simulink model "ModeInputHandle"  (R2018b)
settings: Solver=FixedStepDiscrete  StartTime=0.0  StopTime=10.0  FixedStep=0.01  RelTol=1e-3
undefined symbols (not defined in the file or in its folder): c, CmprtMdHMIReqExt2Tp1, CmprtMdHMIReqExtTp1, CmprtMdHMIReqTp1, d, e, EZESwReq1, f, g, IfVeSMSeStNumConfig, j, KeSMSuButtonLongPressedThrshldTm_Val, KeSMSuFoldType_Val, KeSMSwSeatSMSSeatMdTrigGapTimer_Val, KeSMSwSeatTrigWaitTimer_Val, KeSMSwSRSActiveValidTm_Val, LckUlckActvtFunc1, LstLckFunc1, LugSelectSw1, MdReqTp1, PowerMode1, SeatOccupiedSts1, SRSMode1, StPassCmprtMdCtrl_Md10_VCUConfig_Val, StPassCmprtMdCtrl_Md11_VCUConfig_Val, StPassCmprtMdCtrl_Md12_VCUConfig_Val, StPassCmprtMdCtrl_Md13_VCUConfig_Val, StPassCmprtMdCtrl_Md1_VCUConfig_Val, StPassCmprtMdCtrl_Md27_VCUConfig_Val, StPassCmprtMdCtrl_Md28_VCUConfig_Val, StPassCmprtMdCtrl_Md29_VCUConfig_Val, StPassCmprtMdCtrl_Md2_VCUConfig_Val, StPassCmprtMdCtrl_Md30_VCUConfig_Val, StPassCmprtMdCtrl_Md31_VCUConfig_Val, StPassCmprtMdCtrl_Md32_VCUConfig_Val, StPassCmprtMdCtrl_Md3_VCUConfig_Val, StPassCmprtMdCtrl_Md53_VCUConfig_Val, StPassCmprtMdCtrl_Md56_VCUConfig_Val, StPassCmprtMdCtrl_Md57_VCUConfig_Val, StPassCmprtMdCtrl_Md58_VCUConfig_Val, StPassCmprtMdCtrl_Md61_VCUConfig_Val, StPassCmprtMdCtrl_Md62_VCUConfig_Val, StPassCmprtMdCtrl_Md8_VCUConfig_Val, StPassCmprtMdCtrl_Md9_VCUConfig_Val, StSrv_StMd10_Config_Val, StSrv_StMd11_Config_Val, StSrv_StMd12_Config_Val, StSrv_StMd13_Config_Val, StSrv_StMd1_Config_Val, StSrv_StMd27_Config_Val, StSrv_StMd28_Config_Val, StSrv_StMd29_Config_Val, StSrv_StMd2_Config_Val, StSrv_StMd30_Config_Val, StSrv_StMd31_Config_Val, StSrv_StMd32_Config_Val, StSrv_StMd3_Config_Val, StSrv_StMd8_Config_Val, StSrv_StMd9_Config_Val, VehMovState1
libraries: MSMLib x91
(part 8 of 9)

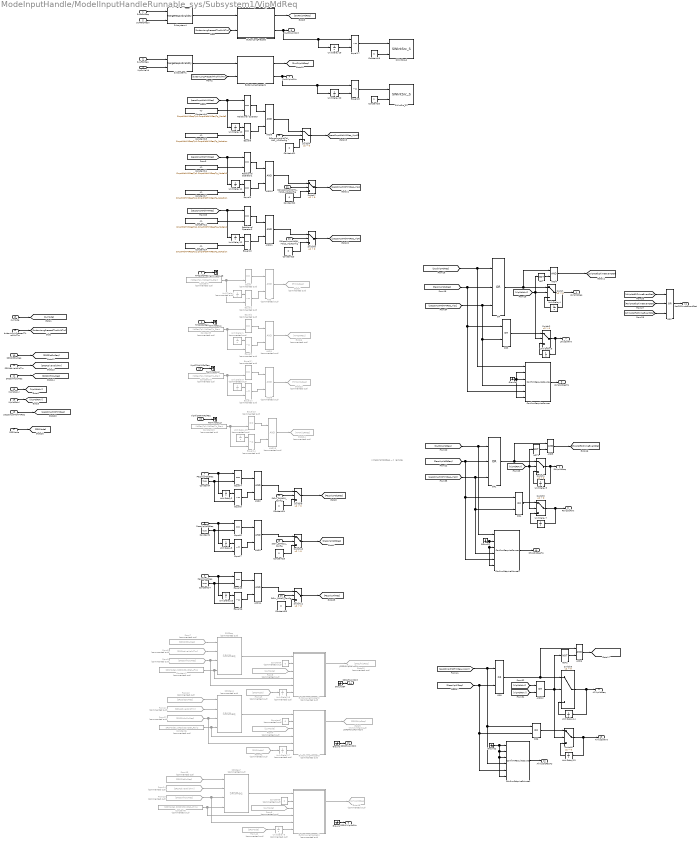
== system ModeInputHandle/ModelInputHandleRunnable_sys/Subsystem1/VipMdReq ==
  note: //SRSLfVipRclIntCnt
  note: // PassVipMdLtReq ---》 remote
  note: //SRSRtVipRclIntCnt
  SwRtRclReq : Inport
  SwRtRclReqV : Inport  Port=2
  SwLfRclReq : Inport  Port=3
  VipSwValid : Inport  Port=4
  HMI2LRclReq : Inport  Port=5
  HMI2RRclReq : Inport  Port=6
  PassVipMdLtReq : Inport  Port=7
  PassVipMdRtReq : Inport  Port=8
  PassVipAllReq : Inport  Port=9
  SRSSlctSwReq : Inport  Port=10
  SRSCnfmSwReq : Inport  Port=11
  buttonLongPressedThrshhldTm : Inport  Port=12
  curMode : Inport  Port=13
  SRSActiveValidTm : Inport  Port=14
  VipMdLtAvl : Inport  Port=15
  VipMdRtAvl : Inport  Port=16
  SRSMode : Inport  Port=17
  passCmprtMdHMIReq : Inport  Port=18
  VipAll2LHMIRclReq : Inport  Port=19
  VipAll2RHMIRclReq : Inport  Port=20
  StPassCmprtMdCtrl_Md10_VCUConfig : Inport  Port=21
  StPassCmprtMdCtrl_Md12_VCUConfig : Inport  Port=22
  StPassCmprtMdCtrl_Md2_VCUConfig : Inport  Port=23
  StSrv_StMd10_Config : Inport  Port=24
  StSrv_StMd12_Config : Inport  Port=25
  StSrv_StMd2_Config : Inport  Port=26
  AND{,1,8,13} (4 alike) : Logic  Commented=on  AllPortsSameDT=off  OutDataTypeStr=boolean
  AND{2..6,9..11,14} (9 alike) : Logic  AllPortsSameDT=off  OutDataTypeStr=boolean
  AND12 : Logic  Operator=OR  AllPortsSameDT=off  OutDataTypeStr=boolean
  ButtonLongPressed : Subsystem  AncestorBlock=MSMLib/ButtonLongPressed
  ButtonLongPressed1 : Subsystem  AncestorBlock=MSMLib/ButtonLongPressed
  ButtonLongPressed2 : Subsystem  Commented=on  AncestorBlock=MSMLib/ButtonLongPressed
  ButtonLongPressed3 : Subsystem  Commented=on  AncestorBlock=MSMLib/ButtonLongPressed
  ButtonLongPressed4 : Subsystem  Commented=on  AncestorBlock=MSMLib/ButtonLongPressed
  ConfirmRequireSource : MSMLib/ConfirmRequireSource  SystemSampleTime=-1
  ConfirmRequireSource1 : MSMLib/ConfirmRequireSource  SystemSampleTime=-1
  ConfirmRequireSource2 : MSMLib/ConfirmRequireSource  SystemSampleTime=-1
  Constant{,3,13,16} (4 alike) : Constant  Commented=on  Value=MdReqTp1.MdReqTp_Start
  Constant1 : Constant  Value=true  OutDataTypeStr=boolean
  Constant10 : Constant  Value=CmprtMdHMIReqTp1.CmprtMdHMIReqTp_Mode2  OutDataTypeStr=Enum:CmprtMdHMIReqTp1
  Constant11 : Constant  Value=CmprtMdHMIReqTp1.CmprtMdHMIReqTp_Mode10  OutDataTypeStr=Enum:CmprtMdHMIReqTp1
  Constant12 : Constant  Value=CmprtMdHMIReqTp1.CmprtMdHMIReqTp_Mode12  OutDataTypeStr=Enum:CmprtMdHMIReqTp1
  Constant14 : Constant  Value=true  OutDataTypeStr=boolean
  Constant15 : Constant  Value=CmprtMdHMIReqTp1.CmprtMdHMIReqTp_NoAction  OutDataTypeStr=Enum:CmprtMdHMIReqTp1
  Constant17 : Constant  Value=CmprtMdHMIReqTp1.CmprtMdHMIReqTp_NoAction  OutDataTypeStr=Enum:CmprtMdHMIReqTp1
  Constant18 : Constant  Value=CmprtMdHMIReqTp1.CmprtMdHMIReqTp_NoAction  OutDataTypeStr=Enum:CmprtMdHMIReqTp1
  Constant19 : Constant  Value=3  OutDataTypeStr=uint8
  Constant2 : Constant  Commented=on  Value=SRSMode1.SRSSlctSwStat_LfVip  OutDataTypeStr=Enum:SRSMode1
  Constant20 : Constant  Value=2  OutDataTypeStr=uint8
  Constant{21..26} (6 alike) : Constant  Value=0  VectorParams1D=off  OutDataTypeStr=boolean  SampleTime=-1
  Constant4 : Constant  Value=true  OutDataTypeStr=boolean
  Constant5 : Constant  Commented=on  Value=0  OutDataTypeStr=uint8
  Constant6 : Constant  Commented=on  Value=SRSMode1.SRSSlctSwStat_RtVip  OutDataTypeStr=Enum:SRSMode1
  Constant7 : Constant  Commented=on  Value=0  OutDataTypeStr=uint8
  Constant8 : Constant  Commented=on  Value=SRSMode1.SRSSlctSwStat_AllVip  OutDataTypeStr=Enum:SRSMode1
  Constant9 : Constant  Commented=on  Value=0  OutDataTypeStr=uint8
  Equal{,2,11,13} (4 alike) : RelationalOperator  Commented=on  Operator===  OutDataTypeStr=boolean  RndMeth=Simplest
  Equal{1,3,12,14} (4 alike) : RelationalOperator  Commented=on  Operator=~=  OutDataTypeStr=boolean  RndMeth=Simplest
  Equal{4,6,8..10,15} (6 alike) : RelationalOperator  Operator===  OutDataTypeStr=boolean  RndMeth=Simplest
  Equal{5,7,16..18} (5 alike) : RelationalOperator  Operator=~=  OutDataTypeStr=boolean  RndMeth=Simplest
  From10 : From  Commented=on  GotoTag=SRSSlctSwReq
  From11 : From  Commented=on  GotoTag=SRSActiveValidTm
  From12 : From  Commented=on  GotoTag=SRSCnfmSwReq
  From13 : From  Commented=on  GotoTag=SRSSlctSwReq
  From14 : From  Commented=on  GotoTag=SRSActiveValidTm
  From15 : From  Commented=on  GotoTag=SRSCnfmSwReq
  From4 : From  Commented=on  GotoTag=curMode
  From40 : From  Commented=on  GotoTag=SRSMode
  From42 : From  Commented=on  GotoTag=SRSMode
  From43 : From  Commented=on  GotoTag=SRSMode
  From5 : From  Commented=on  GotoTag=curMode
  From6 : From  Commented=on  GotoTag=curMode
  From7 : From  Commented=on  GotoTag=SRSSlctSwReq
  From8 : From  Commented=on  GotoTag=SRSActiveValidTm
  From9 : From  Commented=on  GotoTag=SRSCnfmSwReq
  Goto10 : Goto  Commented=on  GotoTag=SRSLfVipReq
  Goto18 : Goto  Commented=on  GotoTag=AllVipMdReq
  Goto23 : Goto  Commented=on  GotoTag=HMIAll2LReq
  Goto24 : Goto  Commented=on  GotoTag=HMIAll2RReq
  Goto6 : Goto  Commented=on  GotoTag=HMI2RReq
  Goto7 : Goto  Commented=on  GotoTag=HMI2LReq
  Goto9 : Goto  Commented=on  GotoTag=SRSRtVipReq
  Ground{,1..4,84} (6 alike) : Ground
  NOT : Logic  Operator=NOT  AllPortsSameDT=off  OutDataTypeStr=boolean
  NOT1 : Logic  Operator=NOT  AllPortsSameDT=off  OutDataTypeStr=boolean
  NOT2 : Logic  Operator=NOT  AllPortsSameDT=off  OutDataTypeStr=boolean
  OR : Logic  Operator=OR  Inputs=3  AllPortsSameDT=off  OutDataTypeStr=boolean
  OR1 : Logic  Operator=OR  Inputs=3  AllPortsSameDT=off  OutDataTypeStr=boolean
  OR2 : Logic  Operator=OR  Inputs=3  AllPortsSameDT=off  OutDataTypeStr=boolean
  OR{3..6} (4 alike) : Logic  Operator=OR  AllPortsSameDT=off  OutDataTypeStr=boolean
  Relational Operator : RelationalOperator  Operator===  OutDataTypeStr=boolean  RndMeth=Simplest
  Relational Operator1 : RelationalOperator  Operator===  OutDataTypeStr=boolean  RndMeth=Simplest
  Relational Operator2 : RelationalOperator  Operator===  OutDataTypeStr=boolean  RndMeth=Simplest
  SRSReq : MSMLib/SRSReq  Commented=on  SystemSampleTime=-1
  SRSReq1 : MSMLib/SRSReq  Commented=on  SystemSampleTime=-1
  SRSReq2 : MSMLib/SRSReq  Commented=on  SystemSampleTime=-1
  SWIntSrc_S : MSMLib/SWIntSrc_S  SystemSampleTime=-1
  SWIntSrc_S1 : MSMLib/SWIntSrc_S  SystemSampleTime=-1
  Subsystem1 : MSMLib/MergeReqAndValidity  SystemSampleTime=-1
  Subsystem4 : MSMLib/MergeReqAndValidity  SystemSampleTime=-1
  Switch{,1..11} (12 alike) : Switch  Criteria=u2 > Threshold
  Terminator_{1..3,69} (4 alike) : Terminator
  Unit Delay{,1,9,15} (4 alike) : UnitDelay  Commented=on  InitialCondition=e  SampleTime=-1
  Unit Delay10 : UnitDelay  InitialCondition=c  SampleTime=-1
  Unit Delay11 : UnitDelay  InitialCondition=c  SampleTime=-1
  Unit Delay12 : UnitDelay  InitialCondition=c  SampleTime=-1
  Unit Delay{2..7,13..14,16,19..20} (11 alike) : UnitDelay  SampleTime=-1
  Unit Delay17 : UnitDelay  Commented=on  InitialCondition=d  SampleTime=-1
  Unit Delay18 : UnitDelay  Commented=on  InitialCondition=d  SampleTime=-1
  Unit Delay8 : UnitDelay  Commented=on  InitialCondition=d  SampleTime=-1
  LtVipMdReq : Outport
  RtVipMdReq : Outport  Port=2
  AllVipMdReq : Outport  Port=3
  SwLfVipIntCnt : Outport  Port=4
  SwRtVipIntCnt : Outport  Port=5
  SRSAllVipIntCnt : Outport  Port=6
  LtVipSoftInt : Outport  Port=7
  RtVipSoftInt : Outport  Port=8
  "LtVipSrcReqTp " : Outport  Port=9
  "RtVipSrcReqTp " : Outport  Port=10
  Notf1ChimeEventStat : Outport  Port=11
  AllVipSrcReqTp : Outport  Port=12
  AllVipSoftInt : Outport  Port=13
  SRSLfVipIntCnt : Outport  Port=14
  SRSRtVipIntCnt : Outport  Port=15
  wires:
  buttonLongPressedThrshhldTm/1 -> [buttonLongPressedThrshhldTm]
  curMode/1 -> [curMode]
  SwRtRclReqV/1 -> Subsystem4/2
  [buttonLongPressedThrshhldTm] -> ButtonLongPressed1/2(longPressThrshhldTm)
  [buttonLongPressedThrshhldTm] -> ButtonLongPressed/2(longPressThrshhldTm)
  SwRtRclReq/1 -> Subsystem4/1
  Subsystem4/1 -> ButtonLongPressed/1(modeReq)
  Equal2/1 -> AND1/1
  Equal1/1 -> AND/2
  AND/1 -> Goto7/1
  Equal/1 -> AND/1
  AND1/1 -> Goto6/1
  Constant3/1 -> Equal3/2, Equal2/2
  Equal3/1 -> AND1/2
  Unit Delay/1 -> Equal1/1
  Unit Delay1/1 -> Equal3/1
  Constant/1 -> Equal1/2, Equal/2
  Constant4/1 -> Equal4/2, Equal5/2
  PassVipMdLtReq/1 -> Unit Delay2/1, Equal4/1
  Equal4/1 -> AND2/1
  Unit Delay2/1 -> Equal5/1
  Equal5/1 -> AND2/2
  Equal7/1 -> AND3/2
  Equal6/1 -> AND3/1
  Unit Delay3/1 -> Equal7/1
  Constant1/1 -> Equal6/2, Equal7/2
  PassVipMdRtReq/1 -> Unit Delay3/1, Equal6/1
  SRSReq/1 -> ButtonLongPressed2/1(modeReq)
  Constant2/1 -> ButtonLongPressed2/4(CmpReq), SRSReq/4
  From5/1 -> ButtonLongPressed2/3(curMdState)
  Constant5/1 -> ButtonLongPressed2/2(longPressThrshhldTm)
  ButtonLongPressed2/1(mdReq) -> Goto10/1
  From4/1 -> ButtonLongPressed3/3(curMdState)
  ButtonLongPressed3/1(mdReq) -> Goto9/1
  SRSReq1/1 -> ButtonLongPressed3/1(modeReq)
  Constant6/1 -> ButtonLongPressed3/4(CmpReq), SRSReq1/4
  Constant7/1 -> ButtonLongPressed3/2(longPressThrshhldTm)
  From6/1 -> ButtonLongPressed4/3(curMdState)
  SRSReq2/1 -> ButtonLongPressed4/1(modeReq)
  Constant8/1 -> ButtonLongPressed4/4(CmpReq), SRSReq2/4
  Constant9/1 -> ButtonLongPressed4/2(longPressThrshhldTm)
  SRSSlctSwReq/1 -> [SRSSlctSwReq]
  SRSActiveValidTm/1 -> [SRSActiveValidTm]
  SRSCnfmSwReq/1 -> [SRSCnfmSwReq]
  From7/1 -> SRSReq/1
  From8/1 -> SRSReq/2
  From9/1 -> ButtonLongPressed2/5(SRSCnfmSwReq), SRSReq/3
  From12/1 -> ButtonLongPressed3/5(SRSCnfmSwReq), SRSReq1/3
  From11/1 -> SRSReq1/2
  From10/1 -> SRSReq1/1
  From15/1 -> ButtonLongPressed4/5(SRSCnfmSwReq), SRSReq2/3
  From14/1 -> SRSReq2/2
  From13/1 -> SRSReq2/1
  ButtonLongPressed/1(mdReq) -> [SwRtVipMdReq]
  ButtonLongPressed1/1(mdReq) -> [SwLfVipMdReq]
  [SwLfVipMdReq] -> OR/1, ConfirmRequireSource/1
  [PassVipMdLtReq] -> OR/2, OR3/1, ConfirmRequireSource/5
  [SwRtVipMdReq] -> OR1/1, ConfirmRequireSource1/1
  [PassVipMdRtReq] -> OR1/2, ConfirmRequireSource1/5, OR4/1
  ConfirmRequireSource/1 -> "LtVipSrcReqTp "/1
  ConfirmRequireSource1/1 -> "RtVipSrcReqTp "/1
  [VipMdLtAvl] -> Switch/2, NOT/1, Switch2/2
  OR/1 -> AND4/1, Switch/1
  Switch/1 -> Unit Delay4/1, LtVipMdReq/1
  Unit Delay4/1 -> Switch/3
  [VipMdRtAvl] -> Switch3/2, NOT1/1, Switch1/2
  OR1/1 -> AND5/1, Switch1/1
  Switch1/1 -> Unit Delay5/1, RtVipMdReq/1
  Unit Delay5/1 -> Switch1/3
  NOT/1 -> AND4/2
  AND4/1 -> [LtVipNotf1ChimeEventStat]
  NOT1/1 -> AND5/2
  AND5/1 -> [RtVipNotf1ChimeEventStat]
  VipMdLtAvl/1 -> [VipMdLtAvl]
  VipMdRtAvl/1 -> [VipMdRtAvl]
  [LtVipNotf1ChimeEventStat] -> OR2/1
  [RtVipNotf1ChimeEventStat] -> OR2/2
  [AllVipNotf1ChimeEventStat] -> OR2/3
  OR2/1 -> Notf1ChimeEventStat/1
  Switch2/1 -> LtVipSoftInt/1, Unit Delay6/1
  Unit Delay6/1 -> Switch2/3
  OR3/1 -> Switch2/1
  Switch3/1 -> RtVipSoftInt/1, Unit Delay7/1
  Unit Delay7/1 -> Switch3/3
  OR4/1 -> Switch3/1
  ButtonLongPressed4/1(mdReq) -> Goto18/1
  Ground/1 -> ConfirmRequireSource/6, ConfirmRequireSource/2, ConfirmRequireSource/3
  Unit Delay8/1 -> ButtonLongPressed4/6(SRSMode)
  Ground1/1 -> ConfirmRequireSource1/6, ConfirmRequireSource1/3, ConfirmRequireSource1/2
  Constant10/1 -> Relational Operator/2
  [passCmprtMdHMIReq] -> Unit Delay10/1, Relational Operator/1
  Equal8/1 -> AND9/2
  Unit Delay10/1 -> Equal8/1
  Relational Operator/1 -> AND9/1
  passCmprtMdHMIReq/1 -> [passCmprtMdHMIReq]
  Equal9/1 -> AND10/2
  Constant11/1 -> Relational Operator1/2
  Relational Operator1/1 -> AND10/1
  [passCmprtMdHMIReq] -> Unit Delay11/1, Relational Operator1/1
  Unit Delay11/1 -> Equal9/1
  Relational Operator2/1 -> AND11/1
  [passCmprtMdHMIReq] -> Unit Delay12/1, Relational Operator2/1
  Unit Delay12/1 -> Equal10/1
  Equal10/1 -> AND11/2
  Constant12/1 -> Relational Operator2/2
  [passCmprtMdHMIReq_VipL] -> OR/3, ConfirmRequireSource/4, OR3/2
  [passCmprtMdHMIReq_VipR] -> ConfirmRequireSource1/4, OR4/2, OR1/3
  [passCmprtMdHMIReq_VipAll] -> OR5/1, ConfirmRequireSource2/4, OR6/1
  ConfirmRequireSource2/1 -> AllVipSrcReqTp/1
  Unit Delay13/1 -> Switch6/3
  Switch5/1 -> Unit Delay14/1, AllVipMdReq/1
  Switch6/1 -> AllVipSoftInt/1, Unit Delay13/1
  Unit Delay14/1 -> Switch5/3
  AND12/1 -> Switch6/2, NOT2/1, Switch5/2
  OR5/1 -> Switch5/1, AND6/1
  [VipMdLtAvl] -> AND12/1
  [VipMdRtAvl] -> AND12/2
  AND8/1 -> Goto23/1
  Equal11/1 -> AND8/1
  Equal12/1 -> AND8/2
  Constant16/1 -> Equal12/2, Equal11/2
  Unit Delay9/1 -> Equal12/1
  OR6/1 -> Switch6/1
  Equal14/1 -> AND13/2
  Unit Delay15/1 -> Equal14/1
  Equal13/1 -> AND13/1
  AND13/1 -> Goto24/1
  Constant13/1 -> Equal14/2, Equal13/2
  Equal15/1 -> AND14/1
  Constant14/1 -> Equal15/2, Equal16/2
  Equal16/1 -> AND14/2
  Unit Delay16/1 -> Equal16/1
  PassVipAllReq/1 -> Unit Delay16/1, Equal15/1
  [PassVipAllReq] -> OR5/2, OR6/2, ConfirmRequireSource2/5
  ButtonLongPressed/2(mdInterruptCnt) -> Unit Delay19/1, Equal17/1, SwRtVipIntCnt/1
  ButtonLongPressed1/2(mdInterruptCnt) -> Unit Delay20/1, Equal18/1, SwLfVipIntCnt/1
  Subsystem1/1 -> ButtonLongPressed1/1(modeReq)
  VipSwValid/1 -> Subsystem1/2
  SwLfRclReq/1 -> Subsystem1/1
  SRSMode/1 -> [SRSMode]
  From40/1 -> Unit Delay8/1
  From42/1 -> Unit Delay17/1
  Unit Delay17/1 -> ButtonLongPressed3/6(SRSMode)
  From43/1 -> Unit Delay18/1
  Unit Delay18/1 -> ButtonLongPressed2/6(SRSMode)
  NOT2/1 -> AND6/2
  AND6/1 -> [AllVipNotf1ChimeEventStat]
  Constant15/1 -> Equal8/2
  Constant17/1 -> Equal9/2
  Constant18/1 -> Equal10/2
  Unit Delay19/1 -> Equal17/2
  Equal17/1 -> SWIntSrc_S/1
  Constant19/1 -> SWIntSrc_S/2
  Unit Delay20/1 -> Equal18/2
  Equal18/1 -> SWIntSrc_S1/1
  Constant20/1 -> SWIntSrc_S1/2
  HMI2LRclReq/1 -> Terminator_69/1
  HMI2RRclReq/1 -> Terminator_1/1
  VipAll2LHMIRclReq/1 -> Terminator_2/1
  VipAll2RHMIRclReq/1 -> Terminator_3/1
  Ground84/1 -> SRSLfVipIntCnt/1
  Ground3/1 -> SRSRtVipIntCnt/1
  Ground4/1 -> SRSAllVipIntCnt/1
  Ground2/1 -> ConfirmRequireSource2/6, ConfirmRequireSource2/3, ConfirmRequireSource2/2, ConfirmRequireSource2/1
  StPassCmprtMdCtrl_Md2_VCUConfig/1 -> Switch4/2
  Constant21/1 -> Switch4/3
  Switch4/1 -> [passCmprtMdHMIReq_VipAll]
  AND9/1 -> Switch4/1
  StPassCmprtMdCtrl_Md10_VCUConfig/1 -> Switch7/2
  AND10/1 -> Switch7/1
  Switch7/1 -> [passCmprtMdHMIReq_VipL]
  Constant22/1 -> Switch7/3
  StPassCmprtMdCtrl_Md12_VCUConfig/1 -> Switch8/2
  AND11/1 -> Switch8/1
  Constant23/1 -> Switch8/3
  Switch8/1 -> [passCmprtMdHMIReq_VipR]
  StSrv_StMd10_Config/1 -> Switch9/2
  AND2/1 -> Switch9/1
  Constant24/1 -> Switch9/3
  Switch9/1 -> [PassVipMdLtReq]
  StSrv_StMd12_Config/1 -> Switch10/2
  AND3/1 -> Switch10/1
  Constant25/1 -> Switch10/3
  Switch10/1 -> [PassVipMdRtReq]
  StSrv_StMd2_Config/1 -> Switch11/2
  AND14/1 -> Switch11/1
  Switch11/1 -> [PassVipAllReq]
  Constant26/1 -> Switch11/3

== system ModeInputHandle/ModelInputHandleRunnable_sys/Subsystem1/WholeVehMem ==
  StPassCmprtMdHMIReqExt2 : Inport
  M61WholeVehMemAvl : Inport  Port=2
  M62WholeVehMemAvl : Inport  Port=3
  StPassCmprtMdCtrl_Md61_VCUConfig : Inport  Port=4
  StPassCmprtMdCtrl_Md62_VCUConfig : Inport  Port=5
  AND{,1..2,10} (4 alike) : Logic  AllPortsSameDT=off  OutDataTypeStr=boolean
  ConfirmRequireSource : MSMLib/ConfirmRequireSource  SystemSampleTime=-1
  ConfirmRequireSource1 : MSMLib/ConfirmRequireSource  SystemSampleTime=-1
  Constant : Constant  Value=0  OutDataTypeStr=boolean
  Constant1 : Constant  Value=CmprtMdHMIReqExt2Tp1.CmprtMdHMIReqExt2Tp_Mode62  OutDataTypeStr=Enum:CmprtMdHMIReqExt2Tp1
  Constant2 : Constant  Value=CmprtMdHMIReqExt2Tp1.CmprtMdHMIReqExt2Tp_NoAction  OutDataTypeStr=Enum:CmprtMdHMIReqExt2Tp1
  Constant3 : Constant  Value=0  OutDataTypeStr=boolean
  Constant4 : Constant  Value=CmprtMdHMIReqExt2Tp1.CmprtMdHMIReqExt2Tp_Mode61  OutDataTypeStr=Enum:CmprtMdHMIReqExt2Tp1
  Constant9 : Constant  Value=CmprtMdHMIReqExt2Tp1.CmprtMdHMIReqExt2Tp_NoAction  OutDataTypeStr=Enum:CmprtMdHMIReqExt2Tp1
  Equal1 : RelationalOperator  Operator===  OutDataTypeStr=boolean  RndMeth=Simplest
  Equal10 : RelationalOperator  Operator===  OutDataTypeStr=boolean  RndMeth=Simplest
  Ground : Ground
  Ground1 : Ground
  NOT : Logic  Operator=NOT  AllPortsSameDT=off  OutDataTypeStr=boolean
  NOT1 : Logic  Operator=NOT  AllPortsSameDT=off  OutDataTypeStr=boolean
  Relational Operator1 : RelationalOperator  Operator===  OutDataTypeStr=boolean  RndMeth=Simplest
  Relational Operator3 : RelationalOperator  Operator===  OutDataTypeStr=boolean  RndMeth=Simplest
  Switch{,1..5} (6 alike) : Switch  Criteria=u2 > Threshold
  Unit Delay{,2..3,6} (4 alike) : UnitDelay  SampleTime=-1
  Unit Delay1 : UnitDelay  InitialCondition=j  SampleTime=-1
  Unit Delay12 : UnitDelay  InitialCondition=j  SampleTime=-1
  WholeVehMem1Req : Outport  VectorParamsAs1DForOutWhenUnconnected=on
  WholeVehMem1srcReqTp : Outport  Port=2  VectorParamsAs1DForOutWhenUnconnected=on
  WholeVehMem1SoftInt : Outport  Port=3
  WholeVehMem1Notf1ChimeEventStat : Outport  Port=4
  WholeVehMem2Req : Outport  Port=5  VectorParamsAs1DForOutWhenUnconnected=on
  WholeVehMem2srcReqTp : Outport  Port=6  VectorParamsAs1DForOutWhenUnconnected=on
  WholeVehMem2SoftInt : Outport  Port=7
  WholeVehMem2Notf1ChimeEventStat : Outport  Port=8
  wires:
  M62WholeVehMemAvl/1 -> Switch3/2, NOT1/1, Switch4/2
  Switch3/1 -> WholeVehMem2Req/1, Unit Delay2/1
  Switch4/1 -> Unit Delay3/1, WholeVehMem2SoftInt/1
  Unit Delay3/1 -> Switch4/3
  NOT1/1 -> AND2/2
  Unit Delay2/1 -> Switch3/3
  AND2/1 -> WholeVehMem2Notf1ChimeEventStat/1
  Ground1/1 -> ConfirmRequireSource1/2, ConfirmRequireSource1/3, ConfirmRequireSource1/6, ConfirmRequireSource1/5, ConfirmRequireSource1/1
  [passCmprtMdHMIReq_WholeVehMem2] -> AND2/1, Switch3/1, ConfirmRequireSource1/4, Switch4/1
  ConfirmRequireSource1/1 -> WholeVehMem2srcReqTp/1
  [StPassCmprtMdHMIReqExt2] -> Relational Operator3/1, Unit Delay12/1
  StPassCmprtMdHMIReqExt2/1 -> [StPassCmprtMdHMIReqExt2]
  Relational Operator1/1 -> AND1/1
  Unit Delay1/1 -> Equal1/1
  Equal1/1 -> AND1/2
  Constant2/1 -> Equal1/2
  Constant1/1 -> Relational Operator1/2
  [StPassCmprtMdHMIReqExt2] -> Relational Operator1/1, Unit Delay1/1
  M61WholeVehMemAvl/1 -> Switch1/2, NOT/1, Switch2/2
  Ground/1 -> ConfirmRequireSource/2, ConfirmRequireSource/3, ConfirmRequireSource/6, ConfirmRequireSource/5, ConfirmRequireSource/1
  ConfirmRequireSource/1 -> WholeVehMem1srcReqTp/1
  AND/1 -> WholeVehMem1Notf1ChimeEventStat/1
  [passCmprtMdHMIReq_WholeVehMem1] -> AND/1, Switch1/1, ConfirmRequireSource/4, Switch2/1
  Switch2/1 -> Unit Delay6/1, WholeVehMem1SoftInt/1
  Unit Delay6/1 -> Switch2/3
  NOT/1 -> AND/2
  Unit Delay/1 -> Switch1/3
  Switch1/1 -> WholeVehMem1Req/1, Unit Delay/1
  Relational Operator3/1 -> AND10/1
  Equal10/1 -> AND10/2
  Constant9/1 -> Equal10/2
  Constant4/1 -> Relational Operator3/2
  Unit Delay12/1 -> Equal10/1
  StPassCmprtMdCtrl_Md61_VCUConfig/1 -> Switch/2
  AND10/1 -> Switch/1
  Switch/1 -> [passCmprtMdHMIReq_WholeVehMem1]
  Constant/1 -> Switch/3
  AND1/1 -> Switch5/1
  StPassCmprtMdCtrl_Md62_VCUConfig/1 -> Switch5/2
  Constant3/1 -> Switch5/3
  Switch5/1 -> [passCmprtMdHMIReq_WholeVehMem2]

== system ModeInputHandle/ModelInputHandleRunnable_sys/Subsystem1/AcsEntry4s2LMdReq/ButtonLongPressed2 ==
  modeReq : Inport
  longPressThrshhldTm : Inport  Port=2
  curMdState : Inport  Port=3
  CmpReq : Inport  Port=4
  SRSCnfmSwReq : Inport  Port=5
  SRSMode : Inport  Port=6
  Chart1 : Stateflow chart  TreatAsAtomicUnit=on
  mdReq : Outport
  mdInterruptCnt : Outport  Port=2
  wires:
  curMdState/1 -> Chart1/3(iCurMdState)
  modeReq/1 -> Chart1/1(iSrc)
  Chart1/1(oMdReq) -> mdReq/1
  Chart1/2(oMdInterruptCnt) -> mdInterruptCnt/1
  longPressThrshhldTm/1 -> Chart1/2(iLongPressThrshhldTm)
  CmpReq/1 -> Chart1/4(iCmpReq)
  SRSCnfmSwReq/1 -> Chart1/5(iCnfmSwReq)
  SRSMode/1 -> Chart1/6(iSRSMode)

== system ModeInputHandle/ModelInputHandleRunnable_sys/Subsystem1/AcsEntry4s2LMdReq/ButtonLongPressed3 ==
  modeReq : Inport
  longPressThrshhldTm : Inport  Port=2
  Chart1 : Stateflow chart  TreatAsAtomicUnit=on
  mdReq : Outport
  mdInterruptCnt : Outport  Port=2
  wires:
  longPressThrshhldTm/1 -> Chart1/2(iLongPressThrshhldTm)
  Chart1/2(oMdInterruptCnt) -> mdInterruptCnt/1
  Chart1/1(oMdReq) -> mdReq/1
  modeReq/1 -> Chart1/1(iSrc)

== system ModeInputHandle/ModelInputHandleRunnable_sys/Subsystem1/AcsEntry4s2RMdReq /ButtonLongPressed ==
  modeReq : Inport
  longPressThrshhldTm : Inport  Port=2
  Chart1 : Stateflow chart  TreatAsAtomicUnit=on
  mdReq : Outport
  mdInterruptCnt : Outport  Port=2
  wires:
  modeReq/1 -> Chart1/1(iSrc)
  Chart1/1(oMdReq) -> mdReq/1
  Chart1/2(oMdInterruptCnt) -> mdInterruptCnt/1
  longPressThrshhldTm/1 -> Chart1/2(iLongPressThrshhldTm)

== system ModeInputHandle/ModelInputHandleRunnable_sys/Subsystem1/AcsEntry4s2RMdReq /ButtonLongPressed2 ==
  modeReq : Inport
  longPressThrshhldTm : Inport  Port=2
  curMdState : Inport  Port=3
  CmpReq : Inport  Port=4
  SRSCnfmSwReq : Inport  Port=5
  SRSMode : Inport  Port=6
  Chart1 : Stateflow chart  TreatAsAtomicUnit=on
  mdReq : Outport
  mdInterruptCnt : Outport  Port=2
  wires:
  SRSMode/1 -> Chart1/6(iSRSMode)
  SRSCnfmSwReq/1 -> Chart1/5(iCnfmSwReq)
  CmpReq/1 -> Chart1/4(iCmpReq)
  longPressThrshhldTm/1 -> Chart1/2(iLongPressThrshhldTm)
  Chart1/2(oMdInterruptCnt) -> mdInterruptCnt/1
  Chart1/1(oMdReq) -> mdReq/1
  modeReq/1 -> Chart1/1(iSrc)
  curMdState/1 -> Chart1/3(iCurMdState)

== system ModeInputHandle/ModelInputHandleRunnable_sys/Subsystem1/AcsEntryMdReq/ButtonLongPressed1 ==
  modeReq : Inport
  longPressThrshhldTm : Inport  Port=2
  Chart1 : Stateflow chart  TreatAsAtomicUnit=on
  mdReq : Outport
  mdInterruptCnt : Outport  Port=2
  wires:
  modeReq/1 -> Chart1/1(iSrc)
  Chart1/1(oMdReq) -> mdReq/1
  Chart1/2(oMdInterruptCnt) -> mdInterruptCnt/1
  longPressThrshhldTm/1 -> Chart1/2(iLongPressThrshhldTm)

== system ModeInputHandle/ModelInputHandleRunnable_sys/Subsystem1/AcsEntryMdReq/ButtonLongPressed2 ==
  modeReq : Inport
  longPressThrshhldTm : Inport  Port=2
  curMdState : Inport  Port=3
  CmpReq : Inport  Port=4
  SRSCnfmSwReq : Inport  Port=5
  SRSMode : Inport  Port=6
  Chart1 : Stateflow chart  TreatAsAtomicUnit=on
  mdReq : Outport
  mdInterruptCnt : Outport  Port=2
  wires:
  curMdState/1 -> Chart1/3(iCurMdState)
  modeReq/1 -> Chart1/1(iSrc)
  Chart1/1(oMdReq) -> mdReq/1
  Chart1/2(oMdInterruptCnt) -> mdInterruptCnt/1
  longPressThrshhldTm/1 -> Chart1/2(iLongPressThrshhldTm)
  CmpReq/1 -> Chart1/4(iCmpReq)
  SRSCnfmSwReq/1 -> Chart1/5(iCnfmSwReq)
  SRSMode/1 -> Chart1/6(iSRSMode)

== system ModeInputHandle/ModelInputHandleRunnable_sys/Subsystem1/AcsEntryMdReq/ButtonLongPressed3 ==
  modeReq : Inport
  longPressThrshhldTm : Inport  Port=2
  Chart1 : Stateflow chart  TreatAsAtomicUnit=on
  mdReq : Outport
  mdInterruptCnt : Outport  Port=2
  wires:
  modeReq/1 -> Chart1/1(iSrc)
  Chart1/1(oMdReq) -> mdReq/1
  Chart1/2(oMdInterruptCnt) -> mdInterruptCnt/1
  longPressThrshhldTm/1 -> Chart1/2(iLongPressThrshhldTm)

== system ModeInputHandle/ModelInputHandleRunnable_sys/Subsystem1/AcsEntryMdReq/ButtonLongPressed4 ==
  modeReq : Inport
  longPressThrshhldTm : Inport  Port=2
  Chart1 : Stateflow chart  TreatAsAtomicUnit=on
  mdReq : Outport
  mdInterruptCnt : Outport  Port=2
  wires:
  modeReq/1 -> Chart1/1(iSrc)
  Chart1/1(oMdReq) -> mdReq/1
  Chart1/2(oMdInterruptCnt) -> mdInterruptCnt/1
  longPressThrshhldTm/1 -> Chart1/2(iLongPressThrshhldTm)

== system ModeInputHandle/ModelInputHandleRunnable_sys/Subsystem1/AcsExit4s2LMdReq/ButtonLongPressed2 ==
  modeReq : Inport
  longPressThrshhldTm : Inport  Port=2
  curMdState : Inport  Port=3
  CmpReq : Inport  Port=4
  SRSCnfmSwReq : Inport  Port=5
  SRSMode : Inport  Port=6
  Chart1 : Stateflow chart  TreatAsAtomicUnit=on
  mdReq : Outport
  mdInterruptCnt : Outport  Port=2
  wires:
  SRSMode/1 -> Chart1/6(iSRSMode)
  SRSCnfmSwReq/1 -> Chart1/5(iCnfmSwReq)
  CmpReq/1 -> Chart1/4(iCmpReq)
  longPressThrshhldTm/1 -> Chart1/2(iLongPressThrshhldTm)
  Chart1/2(oMdInterruptCnt) -> mdInterruptCnt/1
  Chart1/1(oMdReq) -> mdReq/1
  modeReq/1 -> Chart1/1(iSrc)
  curMdState/1 -> Chart1/3(iCurMdState)

== system ModeInputHandle/ModelInputHandleRunnable_sys/Subsystem1/AcsExit4s2LMdReq/ButtonLongPressed3 ==
  modeReq : Inport
  longPressThrshhldTm : Inport  Port=2
  Chart1 : Stateflow chart  TreatAsAtomicUnit=on
  mdReq : Outport
  mdInterruptCnt : Outport  Port=2
  wires:
  modeReq/1 -> Chart1/1(iSrc)
  Chart1/1(oMdReq) -> mdReq/1
  Chart1/2(oMdInterruptCnt) -> mdInterruptCnt/1
  longPressThrshhldTm/1 -> Chart1/2(iLongPressThrshhldTm)

== system ModeInputHandle/ModelInputHandleRunnable_sys/Subsystem1/AcsExit4s2RMdReq/ButtonLongPressed ==
  modeReq : Inport
  longPressThrshhldTm : Inport  Port=2
  Chart1 : Stateflow chart  TreatAsAtomicUnit=on
  mdReq : Outport
  mdInterruptCnt : Outport  Port=2
  wires:
  longPressThrshhldTm/1 -> Chart1/2(iLongPressThrshhldTm)
  Chart1/2(oMdInterruptCnt) -> mdInterruptCnt/1
  Chart1/1(oMdReq) -> mdReq/1
  modeReq/1 -> Chart1/1(iSrc)

== system ModeInputHandle/ModelInputHandleRunnable_sys/Subsystem1/AcsExit4s2RMdReq/ButtonLongPressed2 ==
  modeReq : Inport
  longPressThrshhldTm : Inport  Port=2
  curMdState : Inport  Port=3
  CmpReq : Inport  Port=4
  SRSCnfmSwReq : Inport  Port=5
  SRSMode : Inport  Port=6
  Chart1 : Stateflow chart  TreatAsAtomicUnit=on
  mdReq : Outport
  mdInterruptCnt : Outport  Port=2
  wires:
  curMdState/1 -> Chart1/3(iCurMdState)
  modeReq/1 -> Chart1/1(iSrc)
  Chart1/1(oMdReq) -> mdReq/1
  Chart1/2(oMdInterruptCnt) -> mdInterruptCnt/1
  longPressThrshhldTm/1 -> Chart1/2(iLongPressThrshhldTm)
  CmpReq/1 -> Chart1/4(iCmpReq)
  SRSCnfmSwReq/1 -> Chart1/5(iCnfmSwReq)
  SRSMode/1 -> Chart1/6(iSRSMode)

== system ModeInputHandle/ModelInputHandleRunnable_sys/Subsystem1/AcsExtMdReq/ButtonLongPressed ==
  modeReq : Inport
  longPressThrshhldTm : Inport  Port=2
  Chart1 : Stateflow chart  TreatAsAtomicUnit=on
  mdReq : Outport
  mdInterruptCnt : Outport  Port=2
  wires:
  modeReq/1 -> Chart1/1(iSrc)
  Chart1/1(oMdReq) -> mdReq/1
  Chart1/2(oMdInterruptCnt) -> mdInterruptCnt/1
  longPressThrshhldTm/1 -> Chart1/2(iLongPressThrshhldTm)

== system ModeInputHandle/ModelInputHandleRunnable_sys/Subsystem1/AcsExtMdReq/ButtonLongPressed1 ==
  modeReq : Inport
  longPressThrshhldTm : Inport  Port=2
  Chart1 : Stateflow chart  TreatAsAtomicUnit=on
  mdReq : Outport
  mdInterruptCnt : Outport  Port=2
  wires:
  modeReq/1 -> Chart1/1(iSrc)
  Chart1/1(oMdReq) -> mdReq/1
  Chart1/2(oMdInterruptCnt) -> mdInterruptCnt/1
  longPressThrshhldTm/1 -> Chart1/2(iLongPressThrshhldTm)

== system ModeInputHandle/ModelInputHandleRunnable_sys/Subsystem1/AcsExtMdReq/ButtonLongPressed2 ==
  modeReq : Inport
  longPressThrshhldTm : Inport  Port=2
  curMdState : Inport  Port=3
  CmpReq : Inport  Port=4
  SRSCnfmSwReq : Inport  Port=5
  SRSMode : Inport  Port=6
  Chart1 : Stateflow chart  TreatAsAtomicUnit=on
  mdReq : Outport
  mdInterruptCnt : Outport  Port=2
  wires:
  curMdState/1 -> Chart1/3(iCurMdState)
  modeReq/1 -> Chart1/1(iSrc)
  Chart1/1(oMdReq) -> mdReq/1
  Chart1/2(oMdInterruptCnt) -> mdInterruptCnt/1
  longPressThrshhldTm/1 -> Chart1/2(iLongPressThrshhldTm)
  CmpReq/1 -> Chart1/4(iCmpReq)
  SRSCnfmSwReq/1 -> Chart1/5(iCnfmSwReq)
  SRSMode/1 -> Chart1/6(iSRSMode)

== system ModeInputHandle/ModelInputHandleRunnable_sys/Subsystem1/FamilyMdReq/ButtonLongPressed2 ==
  modeReq : Inport
  longPressThrshhldTm : Inport  Port=2
  curMdState : Inport  Port=3
  CmpReq : Inport  Port=4
  SRSCnfmSwReq : Inport  Port=5
  SRSMode : Inport  Port=6
  Chart1 : Stateflow chart  TreatAsAtomicUnit=on
  mdReq : Outport
  mdInterruptCnt : Outport  Port=2
  wires:
  SRSMode/1 -> Chart1/6(iSRSMode)
  SRSCnfmSwReq/1 -> Chart1/5(iCnfmSwReq)
  CmpReq/1 -> Chart1/4(iCmpReq)
  longPressThrshhldTm/1 -> Chart1/2(iLongPressThrshhldTm)
  Chart1/2(oMdInterruptCnt) -> mdInterruptCnt/1
  Chart1/1(oMdReq) -> mdReq/1
  modeReq/1 -> Chart1/1(iSrc)
  curMdState/1 -> Chart1/3(iCurMdState)

== system ModeInputHandle/ModelInputHandleRunnable_sys/Subsystem1/FamilyMdReq/ButtonLongPressed4 ==
  modeReq : Inport
  longPressThrshhldTm : Inport  Port=2
  curMdState : Inport  Port=3
  CmpReq : Inport  Port=4
  SRSCnfmSwReq : Inport  Port=5
  SRSMode : Inport  Port=6
  Chart1 : Stateflow chart  TreatAsAtomicUnit=on
  mdReq : Outport
  mdInterruptCnt : Outport  Port=2
  wires:
  SRSMode/1 -> Chart1/6(iSRSMode)
  SRSCnfmSwReq/1 -> Chart1/5(iCnfmSwReq)
  CmpReq/1 -> Chart1/4(iCmpReq)
  longPressThrshhldTm/1 -> Chart1/2(iLongPressThrshhldTm)
  Chart1/2(oMdInterruptCnt) -> mdInterruptCnt/1
  Chart1/1(oMdReq) -> mdReq/1
  modeReq/1 -> Chart1/1(iSrc)
  curMdState/1 -> Chart1/3(iCurMdState)

== system ModeInputHandle/ModelInputHandleRunnable_sys/Subsystem1/IntimacyReq/ButtonLongPressed1 ==
  modeReq : Inport
  longPressThrshhldTm : Inport  Port=2
  curMdState : Inport  Port=3
  CmpReq : Inport  Port=4
  SRSCnfmSwReq : Inport  Port=5
  SRSMode : Inport  Port=6
  Chart1 : Stateflow chart  TreatAsAtomicUnit=on
  mdReq : Outport
  mdInterruptCnt : Outport  Port=2
  wires:
  SRSMode/1 -> Chart1/6(iSRSMode)
  SRSCnfmSwReq/1 -> Chart1/5(iCnfmSwReq)
  CmpReq/1 -> Chart1/4(iCmpReq)
  longPressThrshhldTm/1 -> Chart1/2(iLongPressThrshhldTm)
  Chart1/2(oMdInterruptCnt) -> mdInterruptCnt/1
  Chart1/1(oMdReq) -> mdReq/1
  modeReq/1 -> Chart1/1(iSrc)
  curMdState/1 -> Chart1/3(iCurMdState)

== system ModeInputHandle/ModelInputHandleRunnable_sys/Subsystem1/IntimacyReq/ButtonLongPressed4 ==
  modeReq : Inport
  longPressThrshhldTm : Inport  Port=2
  curMdState : Inport  Port=3
  CmpReq : Inport  Port=4
  SRSCnfmSwReq : Inport  Port=5
  SRSMode : Inport  Port=6
  Chart1 : Stateflow chart  TreatAsAtomicUnit=on
  mdReq : Outport
  mdInterruptCnt : Outport  Port=2
  wires:
  SRSMode/1 -> Chart1/6(iSRSMode)
  SRSCnfmSwReq/1 -> Chart1/5(iCnfmSwReq)
  CmpReq/1 -> Chart1/4(iCmpReq)
  longPressThrshhldTm/1 -> Chart1/2(iLongPressThrshhldTm)
  Chart1/2(oMdInterruptCnt) -> mdInterruptCnt/1
  Chart1/1(oMdReq) -> mdReq/1
  modeReq/1 -> Chart1/1(iSrc)
  curMdState/1 -> Chart1/3(iCurMdState)

== system ModeInputHandle/ModelInputHandleRunnable_sys/Subsystem1/LgrstLtMdReq/ButtonLongPressed2 ==
  modeReq : Inport
  longPressThrshhldTm : Inport  Port=2
  curMdState : Inport  Port=3
  CmpReq : Inport  Port=4
  SRSCnfmSwReq : Inport  Port=5
  SRSMode : Inport  Port=6
  Chart1 : Stateflow chart  TreatAsAtomicUnit=on
  mdReq : Outport
  mdInterruptCnt : Outport  Port=2
  wires:
  SRSMode/1 -> Chart1/6(iSRSMode)
  SRSCnfmSwReq/1 -> Chart1/5(iCnfmSwReq)
  CmpReq/1 -> Chart1/4(iCmpReq)
  longPressThrshhldTm/1 -> Chart1/2(iLongPressThrshhldTm)
  Chart1/2(oMdInterruptCnt) -> mdInterruptCnt/1
  Chart1/1(oMdReq) -> mdReq/1
  modeReq/1 -> Chart1/1(iSrc)
  curMdState/1 -> Chart1/3(iCurMdState)

== system ModeInputHandle/ModelInputHandleRunnable_sys/Subsystem1/LgrstLtMdReq/ButtonLongPressed4 ==
  modeReq : Inport
  longPressThrshhldTm : Inport  Port=2
  curMdState : Inport  Port=3
  CmpReq : Inport  Port=4
  SRSCnfmSwReq : Inport  Port=5
  SRSMode : Inport  Port=6
  Chart1 : Stateflow chart  TreatAsAtomicUnit=on
  mdReq : Outport
  mdInterruptCnt : Outport  Port=2
  wires:
  SRSMode/1 -> Chart1/6(iSRSMode)
  SRSCnfmSwReq/1 -> Chart1/5(iCnfmSwReq)
  CmpReq/1 -> Chart1/4(iCmpReq)
  longPressThrshhldTm/1 -> Chart1/2(iLongPressThrshhldTm)
  Chart1/2(oMdInterruptCnt) -> mdInterruptCnt/1
  Chart1/1(oMdReq) -> mdReq/1
  modeReq/1 -> Chart1/1(iSrc)
  curMdState/1 -> Chart1/3(iCurMdState)

== system ModeInputHandle/ModelInputHandleRunnable_sys/Subsystem1/LgrstRtMdReq/ButtonLongPressed2 ==
  modeReq : Inport
  longPressThrshhldTm : Inport  Port=2
  curMdState : Inport  Port=3
  CmpReq : Inport  Port=4
  SRSCnfmSwReq : Inport  Port=5
  SRSMode : Inport  Port=6
  Chart1 : Stateflow chart  TreatAsAtomicUnit=on
  mdReq : Outport
  mdInterruptCnt : Outport  Port=2
  wires:
  SRSMode/1 -> Chart1/6(iSRSMode)
  SRSCnfmSwReq/1 -> Chart1/5(iCnfmSwReq)
  CmpReq/1 -> Chart1/4(iCmpReq)
  longPressThrshhldTm/1 -> Chart1/2(iLongPressThrshhldTm)
  Chart1/2(oMdInterruptCnt) -> mdInterruptCnt/1
  Chart1/1(oMdReq) -> mdReq/1
  modeReq/1 -> Chart1/1(iSrc)
  curMdState/1 -> Chart1/3(iCurMdState)

== system ModeInputHandle/ModelInputHandleRunnable_sys/Subsystem1/LgrstRtMdReq/ButtonLongPressed4 ==
  modeReq : Inport
  longPressThrshhldTm : Inport  Port=2
  curMdState : Inport  Port=3
  CmpReq : Inport  Port=4
  SRSCnfmSwReq : Inport  Port=5
  SRSMode : Inport  Port=6
  Chart1 : Stateflow chart  TreatAsAtomicUnit=on
  mdReq : Outport
  mdInterruptCnt : Outport  Port=2
  wires:
  SRSMode/1 -> Chart1/6(iSRSMode)
  SRSCnfmSwReq/1 -> Chart1/5(iCnfmSwReq)
  CmpReq/1 -> Chart1/4(iCmpReq)
  longPressThrshhldTm/1 -> Chart1/2(iLongPressThrshhldTm)
  Chart1/2(oMdInterruptCnt) -> mdInterruptCnt/1
  Chart1/1(oMdReq) -> mdReq/1
  modeReq/1 -> Chart1/1(iSrc)
  curMdState/1 -> Chart1/3(iCurMdState)

== system ModeInputHandle/ModelInputHandleRunnable_sys/Subsystem1/LugMdReq/ButtonLongPressed ==
  modeReq : Inport
  longPressThrshhldTm : Inport  Port=2
  Chart1 : Stateflow chart  TreatAsAtomicUnit=on
  mdReq : Outport
  mdInterruptCnt : Outport  Port=2
  wires:
  modeReq/1 -> Chart1/1(iSrc)
  Chart1/1(oMdReq) -> mdReq/1
  Chart1/2(oMdInterruptCnt) -> mdInterruptCnt/1
  longPressThrshhldTm/1 -> Chart1/2(iLongPressThrshhldTm)

== system ModeInputHandle/ModelInputHandleRunnable_sys/Subsystem1/LugMdReq/ButtonLongPressed1 ==
  modeReq : Inport
  longPressThrshhldTm : Inport  Port=2
  Chart1 : Stateflow chart  TreatAsAtomicUnit=on
  mdReq : Outport
  mdInterruptCnt : Outport  Port=2
  wires:
  modeReq/1 -> Chart1/1(iSrc)
  Chart1/1(oMdReq) -> mdReq/1
  Chart1/2(oMdInterruptCnt) -> mdInterruptCnt/1
  longPressThrshhldTm/1 -> Chart1/2(iLongPressThrshhldTm)

== system ModeInputHandle/ModelInputHandleRunnable_sys/Subsystem1/LugMdReq/ButtonLongPressed2 ==
  modeReq : Inport
  longPressThrshhldTm : Inport  Port=2
  Chart1 : Stateflow chart  TreatAsAtomicUnit=on
  mdReq : Outport
  mdInterruptCnt : Outport  Port=2
  wires:
  modeReq/1 -> Chart1/1(iSrc)
  Chart1/1(oMdReq) -> mdReq/1
  Chart1/2(oMdInterruptCnt) -> mdInterruptCnt/1
  longPressThrshhldTm/1 -> Chart1/2(iLongPressThrshhldTm)

== system ModeInputHandle/ModelInputHandleRunnable_sys/Subsystem1/LugMdReq/ButtonLongPressed3 ==
  modeReq : Inport
  longPressThrshhldTm : Inport  Port=2
  curMdState : Inport  Port=3
  CmpReq : Inport  Port=4
  SRSCnfmSwReq : Inport  Port=5
  SRSMode : Inport  Port=6
  Chart1 : Stateflow chart  TreatAsAtomicUnit=on
  mdReq : Outport
  mdInterruptCnt : Outport  Port=2
  wires:
  curMdState/1 -> Chart1/3(iCurMdState)
  modeReq/1 -> Chart1/1(iSrc)
  Chart1/1(oMdReq) -> mdReq/1
  Chart1/2(oMdInterruptCnt) -> mdInterruptCnt/1
  longPressThrshhldTm/1 -> Chart1/2(iLongPressThrshhldTm)
  CmpReq/1 -> Chart1/4(iCmpReq)
  SRSCnfmSwReq/1 -> Chart1/5(iCnfmSwReq)
  SRSMode/1 -> Chart1/6(iSRSMode)

== system ModeInputHandle/ModelInputHandleRunnable_sys/Subsystem1/LugMdReq/ButtonLongPressed4 ==
  modeReq : Inport
  longPressThrshhldTm : Inport  Port=2
  curMdState : Inport  Port=3
  CmpReq : Inport  Port=4
  SRSCnfmSwReq : Inport  Port=5
  SRSMode : Inport  Port=6
  Chart1 : Stateflow chart  TreatAsAtomicUnit=on
  mdReq : Outport
  mdInterruptCnt : Outport  Port=2
  wires:
  SRSMode/1 -> Chart1/6(iSRSMode)
  SRSCnfmSwReq/1 -> Chart1/5(iCnfmSwReq)
  CmpReq/1 -> Chart1/4(iCmpReq)
  longPressThrshhldTm/1 -> Chart1/2(iLongPressThrshhldTm)
  Chart1/2(oMdInterruptCnt) -> mdInterruptCnt/1
  Chart1/1(oMdReq) -> mdReq/1
  modeReq/1 -> Chart1/1(iSrc)
  curMdState/1 -> Chart1/3(iCurMdState)

== system ModeInputHandle/ModelInputHandleRunnable_sys/Subsystem1/LugMdReq/ButtonLongPressed5 ==
  modeReq : Inport
  longPressThrshhldTm : Inport  Port=2
  curMdState : Inport  Port=3
  CmpReq : Inport  Port=4
  SRSCnfmSwReq : Inport  Port=5
  SRSMode : Inport  Port=6
  Chart1 : Stateflow chart  TreatAsAtomicUnit=on
  mdReq : Outport
  mdInterruptCnt : Outport  Port=2
  wires:
  curMdState/1 -> Chart1/3(iCurMdState)
  modeReq/1 -> Chart1/1(iSrc)
  Chart1/1(oMdReq) -> mdReq/1
  Chart1/2(oMdInterruptCnt) -> mdInterruptCnt/1
  longPressThrshhldTm/1 -> Chart1/2(iLongPressThrshhldTm)
  CmpReq/1 -> Chart1/4(iCmpReq)
  SRSCnfmSwReq/1 -> Chart1/5(iCnfmSwReq)
  SRSMode/1 -> Chart1/6(iSRSMode)

== system ModeInputHandle/ModelInputHandleRunnable_sys/Subsystem1/LugMdReq/ButtonLongPressed6 ==
  modeReq : Inport
  longPressThrshhldTm : Inport  Port=2
  Chart1 : Stateflow chart  TreatAsAtomicUnit=on
  mdReq : Outport
  mdInterruptCnt : Outport  Port=2
  wires:
  modeReq/1 -> Chart1/1(iSrc)
  Chart1/1(oMdReq) -> mdReq/1
  Chart1/2(oMdInterruptCnt) -> mdInterruptCnt/1
  longPressThrshhldTm/1 -> Chart1/2(iLongPressThrshhldTm)

== system ModeInputHandle/ModelInputHandleRunnable_sys/Subsystem1/LugMdReq/Subsystem1 ==
  src : Inport
  vadility : Inport  Port=2
  Constant : Constant  Value=0  OutDataTypeStr=uint8
  Constant1 : Constant  Value=LugSelectSw1.LugSelectSw_NoAction  OutDataTypeStr=Enum:LugSelectSw1
  Relational Operator : RelationalOperator  Operator===  OutDataTypeStr=boolean  RndMeth=Simplest
  Switch : Switch  Criteria=u2 > Threshold
  req : Outport
  wires:
  vadility/1 -> Relational Operator/1
  Constant/1 -> Relational Operator/2
  Relational Operator/1 -> Switch/2
  src/1 -> Switch/1
  Switch/1 -> req/1
  Constant1/1 -> Switch/3

== system ModeInputHandle/ModelInputHandleRunnable_sys/Subsystem1/LyingMdReq/ButtonLongPressed2 ==
  modeReq : Inport
  longPressThrshhldTm : Inport  Port=2
  curMdState : Inport  Port=3
  CmpReq : Inport  Port=4
  SRSCnfmSwReq : Inport  Port=5
  SRSMode : Inport  Port=6
  Chart1 : Stateflow chart  TreatAsAtomicUnit=on
  mdReq : Outport
  mdInterruptCnt : Outport  Port=2
  wires:
  SRSMode/1 -> Chart1/6(iSRSMode)
  SRSCnfmSwReq/1 -> Chart1/5(iCnfmSwReq)
  CmpReq/1 -> Chart1/4(iCmpReq)
  longPressThrshhldTm/1 -> Chart1/2(iLongPressThrshhldTm)
  Chart1/2(oMdInterruptCnt) -> mdInterruptCnt/1
  Chart1/1(oMdReq) -> mdReq/1
  modeReq/1 -> Chart1/1(iSrc)
  curMdState/1 -> Chart1/3(iCurMdState)

== system ModeInputHandle/ModelInputHandleRunnable_sys/Subsystem1/LyingMdReq/ButtonLongPressed4 ==
  modeReq : Inport
  longPressThrshhldTm : Inport  Port=2
  curMdState : Inport  Port=3
  CmpReq : Inport  Port=4
  SRSCnfmSwReq : Inport  Port=5
  SRSMode : Inport  Port=6
  Chart1 : Stateflow chart  TreatAsAtomicUnit=on
  mdReq : Outport
  mdInterruptCnt : Outport  Port=2
  wires:
  SRSMode/1 -> Chart1/6(iSRSMode)
  SRSCnfmSwReq/1 -> Chart1/5(iCnfmSwReq)
  CmpReq/1 -> Chart1/4(iCmpReq)
  longPressThrshhldTm/1 -> Chart1/2(iLongPressThrshhldTm)
  Chart1/2(oMdInterruptCnt) -> mdInterruptCnt/1
  Chart1/1(oMdReq) -> mdReq/1
  modeReq/1 -> Chart1/1(iSrc)
  curMdState/1 -> Chart1/3(iCurMdState)

== system ModeInputHandle/ModelInputHandleRunnable_sys/Subsystem1/PasReclinerEntryMdReq/ButtonLongPressed ==
  modeReq : Inport
  longPressThrshhldTm : Inport  Port=2
  Chart1 : Stateflow chart  TreatAsAtomicUnit=on
  mdReq : Outport
  mdInterruptCnt : Outport  Port=2
  wires:
  modeReq/1 -> Chart1/1(iSrc)
  Chart1/1(oMdReq) -> mdReq/1
  Chart1/2(oMdInterruptCnt) -> mdInterruptCnt/1
  longPressThrshhldTm/1 -> Chart1/2(iLongPressThrshhldTm)

== system ModeInputHandle/ModelInputHandleRunnable_sys/Subsystem1/PasReclinerExitMdReq/ButtonLongPressed ==
  modeReq : Inport
  longPressThrshhldTm : Inport  Port=2
  Chart1 : Stateflow chart  TreatAsAtomicUnit=on
  mdReq : Outport
  mdInterruptCnt : Outport  Port=2
  wires:
  longPressThrshhldTm/1 -> Chart1/2(iLongPressThrshhldTm)
  Chart1/2(oMdInterruptCnt) -> mdInterruptCnt/1
  Chart1/1(oMdReq) -> mdReq/1
  modeReq/1 -> Chart1/1(iSrc)

== system ModeInputHandle/ModelInputHandleRunnable_sys/Subsystem1/RecoveryMdReq/ButtonLongPressed ==
  modeReq : Inport
  longPressThrshhldTm : Inport  Port=2
  Chart1 : Stateflow chart  TreatAsAtomicUnit=on
  mdReq : Outport
  mdInterruptCnt : Outport  Port=2
  wires:
  modeReq/1 -> Chart1/1(iSrc)
  Chart1/1(oMdReq) -> mdReq/1
  Chart1/2(oMdInterruptCnt) -> mdInterruptCnt/1
  longPressThrshhldTm/1 -> Chart1/2(iLongPressThrshhldTm)

== system ModeInputHandle/ModelInputHandleRunnable_sys/Subsystem1/RecoveryMdReq/ButtonLongPressed1 ==
  modeReq : Inport
  longPressThrshhldTm : Inport  Port=2
  Chart1 : Stateflow chart  TreatAsAtomicUnit=on
  mdReq : Outport
  mdInterruptCnt : Outport  Port=2
  wires:
  modeReq/1 -> Chart1/1(iSrc)
  Chart1/1(oMdReq) -> mdReq/1
  Chart1/2(oMdInterruptCnt) -> mdInterruptCnt/1
  longPressThrshhldTm/1 -> Chart1/2(iLongPressThrshhldTm)

== system ModeInputHandle/ModelInputHandleRunnable_sys/Subsystem1/RecoveryMdReq/ButtonLongPressed2 ==
  modeReq : Inport
  longPressThrshhldTm : Inport  Port=2
  curMdState : Inport  Port=3
  CmpReq : Inport  Port=4
  SRSCnfmSwReq : Inport  Port=5
  SRSMode : Inport  Port=6
  Chart1 : Stateflow chart  TreatAsAtomicUnit=on
  mdReq : Outport
  mdInterruptCnt : Outport  Port=2
  wires:
  SRSMode/1 -> Chart1/6(iSRSMode)
  SRSCnfmSwReq/1 -> Chart1/5(iCnfmSwReq)
  CmpReq/1 -> Chart1/4(iCmpReq)
  longPressThrshhldTm/1 -> Chart1/2(iLongPressThrshhldTm)
  Chart1/2(oMdInterruptCnt) -> mdInterruptCnt/1
  Chart1/1(oMdReq) -> mdReq/1
  modeReq/1 -> Chart1/1(iSrc)
  curMdState/1 -> Chart1/3(iCurMdState)

== system ModeInputHandle/ModelInputHandleRunnable_sys/Subsystem1/RecoveryMdReq/ButtonLongPressed4 ==
  modeReq : Inport
  longPressThrshhldTm : Inport  Port=2
  curMdState : Inport  Port=3
  CmpReq : Inport  Port=4
  SRSCnfmSwReq : Inport  Port=5
  SRSMode : Inport  Port=6
  Chart1 : Stateflow chart  TreatAsAtomicUnit=on
  mdReq : Outport
  mdInterruptCnt : Outport  Port=2
  wires:
  SRSMode/1 -> Chart1/6(iSRSMode)
  SRSCnfmSwReq/1 -> Chart1/5(iCnfmSwReq)
  CmpReq/1 -> Chart1/4(iCmpReq)
  longPressThrshhldTm/1 -> Chart1/2(iLongPressThrshhldTm)
  Chart1/2(oMdInterruptCnt) -> mdInterruptCnt/1
  Chart1/1(oMdReq) -> mdReq/1
  modeReq/1 -> Chart1/1(iSrc)
  curMdState/1 -> Chart1/3(iCurMdState)

== system ModeInputHandle/ModelInputHandleRunnable_sys/Subsystem1/UnfoldMdReq/ButtonLongPressed ==
  modeReq : Inport
  longPressThrshhldTm : Inport  Port=2
  Chart1 : Stateflow chart  TreatAsAtomicUnit=on
  mdReq : Outport
  mdInterruptCnt : Outport  Port=2
  wires:
  modeReq/1 -> Chart1/1(iSrc)
  Chart1/1(oMdReq) -> mdReq/1
  Chart1/2(oMdInterruptCnt) -> mdInterruptCnt/1
  longPressThrshhldTm/1 -> Chart1/2(iLongPressThrshhldTm)

== system ModeInputHandle/ModelInputHandleRunnable_sys/Subsystem1/UnfoldMdReq/ButtonLongPressed1 ==
  modeReq : Inport
  longPressThrshhldTm : Inport  Port=2
  Chart1 : Stateflow chart  TreatAsAtomicUnit=on
  mdReq : Outport
  mdInterruptCnt : Outport  Port=2
  wires:
  modeReq/1 -> Chart1/1(iSrc)
  Chart1/1(oMdReq) -> mdReq/1
  Chart1/2(oMdInterruptCnt) -> mdInterruptCnt/1
  longPressThrshhldTm/1 -> Chart1/2(iLongPressThrshhldTm)

== system ModeInputHandle/ModelInputHandleRunnable_sys/Subsystem1/VipMdReq/ButtonLongPressed ==
  modeReq : Inport
  longPressThrshhldTm : Inport  Port=2
  Chart1 : Stateflow chart  TreatAsAtomicUnit=on
  mdReq : Outport
  mdInterruptCnt : Outport  Port=2
  wires:
  modeReq/1 -> Chart1/1(iSrc)
  Chart1/1(oMdReq) -> mdReq/1
  Chart1/2(oMdInterruptCnt) -> mdInterruptCnt/1
  longPressThrshhldTm/1 -> Chart1/2(iLongPressThrshhldTm)

== system ModeInputHandle/ModelInputHandleRunnable_sys/Subsystem1/VipMdReq/ButtonLongPressed1 ==
  modeReq : Inport
  longPressThrshhldTm : Inport  Port=2
  Chart1 : Stateflow chart  TreatAsAtomicUnit=on
  mdReq : Outport
  mdInterruptCnt : Outport  Port=2
  wires:
  modeReq/1 -> Chart1/1(iSrc)
  Chart1/1(oMdReq) -> mdReq/1
  Chart1/2(oMdInterruptCnt) -> mdInterruptCnt/1
  longPressThrshhldTm/1 -> Chart1/2(iLongPressThrshhldTm)

== system ModeInputHandle/ModelInputHandleRunnable_sys/Subsystem1/VipMdReq/ButtonLongPressed2 ==
  modeReq : Inport
  longPressThrshhldTm : Inport  Port=2
  curMdState : Inport  Port=3
  CmpReq : Inport  Port=4
  SRSCnfmSwReq : Inport  Port=5
  SRSMode : Inport  Port=6
  Chart1 : Stateflow chart  TreatAsAtomicUnit=on
  mdReq : Outport
  mdInterruptCnt : Outport  Port=2
  wires:
  SRSMode/1 -> Chart1/6(iSRSMode)
  SRSCnfmSwReq/1 -> Chart1/5(iCnfmSwReq)
  CmpReq/1 -> Chart1/4(iCmpReq)
  longPressThrshhldTm/1 -> Chart1/2(iLongPressThrshhldTm)
  Chart1/2(oMdInterruptCnt) -> mdInterruptCnt/1
  Chart1/1(oMdReq) -> mdReq/1
  modeReq/1 -> Chart1/1(iSrc)
  curMdState/1 -> Chart1/3(iCurMdState)

== system ModeInputHandle/ModelInputHandleRunnable_sys/Subsystem1/VipMdReq/ButtonLongPressed3 ==
  modeReq : Inport
  longPressThrshhldTm : Inport  Port=2
  curMdState : Inport  Port=3
  CmpReq : Inport  Port=4
  SRSCnfmSwReq : Inport  Port=5
  SRSMode : Inport  Port=6
  Chart1 : Stateflow chart  TreatAsAtomicUnit=on
  mdReq : Outport
  mdInterruptCnt : Outport  Port=2
  wires:
  curMdState/1 -> Chart1/3(iCurMdState)
  modeReq/1 -> Chart1/1(iSrc)
  Chart1/1(oMdReq) -> mdReq/1
  Chart1/2(oMdInterruptCnt) -> mdInterruptCnt/1
  longPressThrshhldTm/1 -> Chart1/2(iLongPressThrshhldTm)
  CmpReq/1 -> Chart1/4(iCmpReq)
  SRSCnfmSwReq/1 -> Chart1/5(iCnfmSwReq)
  SRSMode/1 -> Chart1/6(iSRSMode)

== system ModeInputHandle/ModelInputHandleRunnable_sys/Subsystem1/VipMdReq/ButtonLongPressed4 ==
  modeReq : Inport
  longPressThrshhldTm : Inport  Port=2
  curMdState : Inport  Port=3
  CmpReq : Inport  Port=4
  SRSCnfmSwReq : Inport  Port=5
  SRSMode : Inport  Port=6
  Chart1 : Stateflow chart  TreatAsAtomicUnit=on
  mdReq : Outport
  mdInterruptCnt : Outport  Port=2
  wires:
  curMdState/1 -> Chart1/3(iCurMdState)
  modeReq/1 -> Chart1/1(iSrc)
  Chart1/1(oMdReq) -> mdReq/1
  Chart1/2(oMdInterruptCnt) -> mdInterruptCnt/1
  longPressThrshhldTm/1 -> Chart1/2(iLongPressThrshhldTm)
  CmpReq/1 -> Chart1/4(iCmpReq)
  SRSCnfmSwReq/1 -> Chart1/5(iCnfmSwReq)
  SRSMode/1 -> Chart1/6(iSRSMode)

== stateflow chart ModeInputHandle/ModelInputHandleRunnable_sys/Subsystem1/AcsExit4s2LMdReq/ButtonLongPressed2/Chart1 ==
  state NotPressed
    en:
    oMdReq = false;
  state ButtonPressed
    state idle
    state idle1
      en:
      oMdReq = true;
    (default) -> idle
    idle -> idle1 : [after(iLongPressThrshhldTm,tick)]
  (default) -> NotPressed : {oMdInterruptCnt = 0;}
  NotPressed -> NotPressed [order 1] : [(iSRSMode != SRSCurMode1.SRSMode_None) &&...
      | hasChangedTo(iCnfmSwReq, true)]
      | {oMdInterruptCnt ++;}
  NotPressed -> ButtonPressed [order 2] : [iCurMdState == MdTp1.MdTp_None &&...
      | hasChangedTo(iSrc, true)]
  ButtonPressed -> NotPressed : [!iSrc]
  data: iSrc input boolean; oMdReq output boolean; oMdInterruptCnt output uint8; iLongPressThrshhldTm input uint8; iCurMdState input Enum: MdTp1; iCmpReq input; iCnfmSwReq input boolean; iSRSMode input Enum: SRSCurMode1

== stateflow chart ModeInputHandle/ModelInputHandleRunnable_sys/Subsystem1/AcsExit4s2LMdReq/ButtonLongPressed3/Chart1 ==
  state NotPressed
    en:
    oMdReq = false;
  state ButtonPressed
    state idle
    state idle1
      en:
      oMdReq=true;
    (default) -> idle
    idle -> idle1 [order 2] : [after(iLongPressThrshhldTm,tick)]
  (default) -> NotPressed : {oMdInterruptCnt = 0;}
  NotPressed -> ButtonPressed : [hasChangedTo(iSrc, true)]
  idle -> NotPressed [order 1] : [!iSrc]
      | {oMdInterruptCnt ++;}
  idle1 -> NotPressed : [!iSrc]
  data: iSrc input boolean; oMdReq output boolean; oMdInterruptCnt output uint8; iLongPressThrshhldTm input uint8

== stateflow chart ModeInputHandle/ModelInputHandleRunnable_sys/Subsystem1/AcsEntry4s2LMdReq/ButtonLongPressed2/Chart1 ==
  state NotPressed
    en:
    oMdReq = false;
  state ButtonPressed
    state idle
    state idle1
      en:
      oMdReq = true;
    (default) -> idle
    idle -> idle1 : [after(iLongPressThrshhldTm,tick)]
  (default) -> NotPressed : {oMdInterruptCnt = 0;}
  NotPressed -> NotPressed [order 1] : [(iSRSMode != SRSCurMode1.SRSMode_None) &&...
      | hasChangedTo(iCnfmSwReq, true)]
      | {oMdInterruptCnt ++;}
  NotPressed -> ButtonPressed [order 2] : [iCurMdState == MdTp1.MdTp_None &&...
      | hasChangedTo(iSrc, true)]
  ButtonPressed -> NotPressed : [!iSrc]
  data: iSrc input boolean; oMdReq output boolean; oMdInterruptCnt output uint8; iLongPressThrshhldTm input uint8; iCurMdState input Enum: MdTp1; iCmpReq input; iCnfmSwReq input boolean; iSRSMode input Enum: SRSCurMode1

== stateflow chart ModeInputHandle/ModelInputHandleRunnable_sys/Subsystem1/AcsEntry4s2LMdReq/ButtonLongPressed3/Chart1 ==
  state NotPressed
    en:
    oMdReq = false;
  state ButtonPressed
    state idle
    state idle1
      en:
      oMdReq=true;
    (default) -> idle
    idle -> idle1 [order 2] : [after(iLongPressThrshhldTm,tick)]
  (default) -> NotPressed : {oMdInterruptCnt = 0;}
  NotPressed -> ButtonPressed : [hasChangedTo(iSrc, true)]
  idle -> NotPressed [order 1] : [!iSrc]
      | {oMdInterruptCnt ++;}
  idle1 -> NotPressed : [!iSrc]
  data: iSrc input boolean; oMdReq output boolean; oMdInterruptCnt output uint8; iLongPressThrshhldTm input uint8
